simulink library "MS2G_Parts_Lib"  (R2016a)
settings: Solver=ode45  StartTime=0.0  StopTime=10.0  RelTol=1e-3
undefined symbols (not defined in the file or in its folder): Extr_Data_Link1Hole, Extr_Data_Link2Hole, Extr_Data_Ring, Local, X, Y, Z
libraries: sm_lib x58, MS2G_Parts_Lib x8
(part 1 of 2)
Description:
  | Copyright 2013-2016 The MathWorks, Inc.
settings Model: Creator=smiller  LastModifiedBy=smiller
settings DataIOCC: LimitDataPoints=on  SaveFormat=Array  SignalLoggingSaveFormat=ModelDataLogs
settings OptimizationCC: ExpressionDepthLimit=2147483647
settings DebuggingCC: UnderspecifiedInitializationDetection=Classic  MergeDetectMultiDrivingBlocksExec=none  SolverPrmCheckMsg=warning  FcnCallInpInsideContextMsg=EnableAllAsWarning  StateNameClashWarn=warning
settings HardwareCC: ProdBitPerPointer=32  ProdLargestAtomicFloat=None  ProdIntDivRoundTo=Undefined  ProdEndianess=Unspecified  ProdWordSize=32  ProdHWDeviceType=32-bit Generic
settings ModelReferenceCC: PropagateSignalLabelsOutOfModel=off
settings ConfigComp: CovModelRefEnable=Off

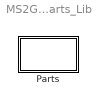
== system MS2G_Parts_Lib ==
  Parts : Subsystem

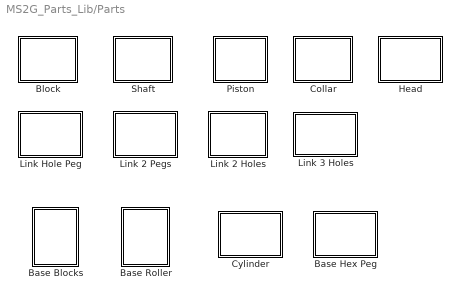
== system MS2G_Parts_Lib/Parts ==
  Base Blocks : Subsystem  mask(Base Blocks){block_length=6, block_width=16, block_height=16, shaft_radius=5, shaft_length=4.4, material_density=1000, material_color=[0 0.6 0.8], material_opacity=1}
      mask prompts: block_length "Length (cm)"; block_width "Width (cm)"; block_height "Height (cm)"; shaft_radius "Radius (cm)"; shaft_length "Length (cm)"; material_density "Density (kg/m^3)"; material_color "Color"; material_opacity "Opacity"
      mask help: Parameterized base with two blocks and a shaft.
      mask Display:
      | image(imread('Base_Blocks_IMAGE.jpg'));
      | port_label('RConn',1,'S');
      | port_label('LConn',1,'B');
  Base Hex Peg : Subsystem  mask(Four bar base body){R=3, T=0.5, rp=0.5, lp=1.5, clr=[0.4 0.4 0.4], img_file=sm_four_bar_base.png}
      mask prompts: R "Base radius (cm):"; T "Base thickeness (cm):"; rp "Peg radius (cm):"; lp "Peg length (cm):"; clr "Base color:"; img_file "Image file:"
      mask help: Base body on the crank side of the four bar mechanism
      mask Display:
      | image(imread('Base_Hex_Peg_IMAGE.jpg'));
      | port_label('LConn',1,'B');
      | port_label('RConn',1,'P');
  Base Roller : Subsystem  mask(Base Roller){roller_length=6, roller_radius=8, shaft_length=4.4, shaft_radius=5, material_density=1000, material_color=[0 0.6 0.8], material_opacity=1}
      mask prompts: roller_length "Length (cm)"; roller_radius "Radius (cm)"; shaft_length "Length (cm)"; shaft_radius "Radius (cm)"; material_density "Density (kg/m^3)"; material_color "Color"; material_opacity "Opacity"
      mask help: Parameterized roller with two wheels connected by a shaft.
      mask Display:
      | image(imread('Base_Roller_IMAGE.jpg'));
      | port_label('RConn',1,'S');
      | port_label('LConn',1,'B');
  Block : Subsystem  mask(Block){L=6, W=16, H=16, z_ori=Local +Z, rho=1000, clr=[0 0.6 0.8], opc=1}
      mask prompts: L "Length (cm):"; W "Width (cm):"; H "Height (cm):"; z_ori "Shaft orientation:"; rho "Shaft density (kg/m^3):"; clr "Link color:"; opc "Opacity:"
      mask help: Rectangular block. Ports are at the center of the faces normal to the local z-axis. Can be configured to have positive Z from B to F or from F to B.
      mask init:
      | if(z_ori == 2)
      |     z_ori = -1;
      | end
      mask TypeOptions z_ori: Local +Z | Local -Z
      mask Display:
      | image(imread('Block_IMAGE.jpg'));
      | port_label('LConn',1,'B');
      | port_label('RConn',1,'F');
  Collar : Subsystem  mask{collar_length=30, collar_radius=6.5, cylinder_length=20, cylinder_radius=6.5, cylinder_ori=Local +Z, material_density=1000, material_color=[0.5 0.5 0.5], material_opacity=1}
      mask prompts: collar_length "Length (cm):"; collar_radius "Radius (cm):"; cylinder_length "Length (cm):"; cylinder_radius "Radius (cm):"; cylinder_ori "Orientation (B to C):"; material_density "Density (kg/m^3):"; material_color "Color:"; material_opacity "Opacity:"
      mask init:
      | if(cylinder_ori == 2)
      |     cylinder_ori = -1;
      | end
      mask TypeOptions cylinder_ori: Local +Z | Local -Z
      mask Display:
      | image(imread('Actuator_Collar_IMAGE.jpg'));
      | port_label('LConn',1,'B');
      | port_label('RConn',1,'C');
  Cylinder : Subsystem  mask(Annular Cylinder){Ro=5, Ri=4, L=6, Ang_Sw=180, cyl_z=-4, cyl_theta=0, cyl_radius=18, rho=100, clr=[0.4 0.4 0.4], opc=0.5}
      mask prompts: Ro "Cylinder outer radius (cm)"; Ri "Cylinder inner radius (cm)"; L "Cylinder length (cm)"; Ang_Sw "Cylinder  sweep angle (deg)"; cyl_z "Z position (cm)"; cyl_theta "Theta (deg)"; cyl_radius "Radius (cm)"; rho "Density (kg/m^3)"; clr "Color"; opc "Opacity"
      mask Display:
      | image(imread('Cylinder_Half_IMAGE.jpg'));
      | port_label('LConn',1,'S')
      | port_label('RConn',1,'R')
  Head : Subsystem  mask(Piston Head){Ro=4, Ri=3, L=5, Rp=0.5, rho=100, clr=[0 1 0], opc=0.5}
      mask prompts: Ro "Cylinder outer radius (cm)"; Ri "Cylinder inner radius (cm)"; L "Cylinder length (cm)"; Rp "Pin radius (cm)"; rho "Density (kg/m^3)"; clr "Color"; opc "Opacity"
      mask help: Piston head with pin for rotating connection to rod. C port is aligned for translational motion in cylinder.
      mask Display:
      | image(imread('Piston_Peg_IMAGE.jpg'));
      | port_label('RConn',1,'C')
      | port_label('LConn',1,'P')
  Link 2 Holes : Subsystem  mask(Connector Link, 2 Holes){L=13, W=2, T=1, r=0.5, rho=10, clr=[0.6 0.6 0.0], opc=1}
      mask prompts: L "Link length (cm):"; W "Link width (cm):"; T "Link thickness (cm):"; r "Hole radius (cm):"; rho "Link density (kg/m^3):"; clr "Link color:"; opc "Opacity"
      mask help: Connector link with two holes. Ports are located at centers of holes, oriented such that Z is out of the hole, positive X is from L hole to R hole.
      mask Display:
      | image(imread('Link_Hole_Hole_IMAGE.jpg'));
      | port_label('LConn',1,'L');
      | port_label('RConn',1,'R');
  Link 2 Pegs : Subsystem  mask(Connector Link, 2 Pegs){L=4.5, W=2, T=0.5, r=0.5, z_ori_l=Local -Z, z_ori_r=Local -Z, Ro=1000, clr=[0.0 0.6 0.8], opc=1}
      mask prompts: L "Link length (cm):"; W "Link width (cm):"; T "Link thickness (cm):"; r "Peg radius (cm):"; z_ori_l "Peg Orientation, Left"; z_ori_r "Peg Orientation, Right"; Ro "Link density (kg/m^3):"; clr "Link color:"; opc "Opacity"
      mask help: Connector link with two pegs. The L and R ports are located at the outward face of each peg, and are oriented such that the Z-axis points along the axis of the peg, and positive X is from the left peg to the right peg. The pegs can be configured to be on the upper or lower side of the link.
      mask init:
      | if(z_ori_l == 2)
      |     z_ori_l = -1;
      | end
      | 
      | if(z_ori_r == 2)
      |     z_ori_r = -1;
      | end
      mask TypeOptions z_ori_l: Local +Z | Local -Z
      mask TypeOptions z_ori_r: Local +Z | Local -Z
      mask Display:
      | image(imread('Link_2Peg_IMAGE.jpg'));
      | port_label('LConn',1,'L');
      | port_label('RConn',1,'R');
  Link 3 Holes : Subsystem  mask(Connector Link, 2 Holes){L=240, W=15, T=4, r=5, rho=1000, clr_string=Yellow, opc=1}
      mask prompts: L "Link length (cm):"; W "Link width (cm):"; T "Link thickness (cm):"; r "Hole radius (cm):"; rho "Link density (kg/m^3):"; clr_string "Link color:"; opc "Opacity:"
      mask help: Connector link with two holes. Ports are located at centers of holes, oriented such that Z is out of the hole, positive X is from L hole to R hole.
      mask init:
      | imgfile='Link_3_Hole_Yellow_IMAGE.jpg';
      | if(strcmp(clr_string,'Yellow'))
      |     clr = [0.6 0.6 0.0];
      | else
      |     clr = [0.8 0.2 0.0];
      |     imgfile='Link_3_Hole_Red_IMAGE.jpg';
      | end
      mask TypeOptions clr_string: Yellow | Red
      mask Display:
      | image(imread(imgfile));
      | port_label('RConn',1,'F');
      | port_label('RConn',2,'C');
      | port_label('RConn',3,'R');
  Link Hole Peg : Subsystem  mask(Connector Link, Hole Peg){L=4.5, W=2, T=1.5, r=0.5, z_ori=Local +Z, Ro=1000, clr=[0.0 0.6 0.8], opc=1}
      mask prompts: L "Link length (cm):"; W "Link width (cm):"; T "Link thickness (cm):"; r "Peg/Hole radius (cm):"; z_ori "Peg Orientation:"; Ro "Link density (kg/m^3):"; clr "Link color:"; opc "Opacity"
      mask help: Connector Link with one hole and one peg. The H port is at the center of the hole. The P port is at the outward face of the peg. Frames are oriented such that Z points out of the hole, positive X is from the hole to the peg. The peg can be placed on the upper or lower side of the link.
      mask init:
      | if(z_ori == 2)
      |     z_ori = -1;
      | end
      mask TypeOptions z_ori: Local +Z | Local -Z
      mask Display:
      | image(imread('Link_Hole_Peg_IMAGE.jpg'));
      | port_label('LConn',1,'H');
      | port_label('RConn',1,'P');
  Piston : Subsystem
      mask Display:
      | image(imread('Piston_Shaft_IMAGE.jpg'));
      | port_label('RConn',1,'P');
      | port_label('LConn',1,'R');
  Shaft : Subsystem  mask(Cylindrical Shaft){L=10, r=5, theta=0, z_ori=Local -Z, Ro=1000, clr=[0.0 0.6 0.8], opc=1}
      mask prompts: L "Length (cm):"; r "Radius (cm):"; theta "Twist (deg)"; z_ori "Orientation (B to F)"; Ro "Density (kg/m^3):"; clr "Color:"; opc "Opacity"
      mask help: Cylindrical shaft. Ports are at shaft ends, and oriented such that the Z-axis is between the ports. Can be configured to have positive Z from B to F or from F to B.
      mask init:
      | if(z_ori == 2)
      |     z_ori = -1;
      | end
      mask TypeOptions z_ori: Local +Z | Local -Z
      mask Display:
      | image(imread('Shaft_IMAGE.jpg'));
      | port_label('LConn',1,'B');
      | port_label('RConn',1,'F');

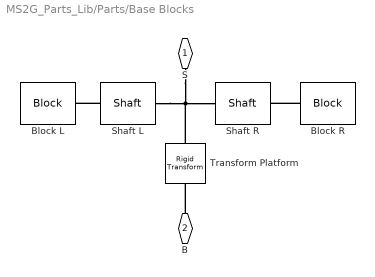
== system MS2G_Parts_Lib/Parts/Base Blocks ==
  Block L : MS2G_Parts_Lib/Parts/Block  L=block_length  W=block_width  H=block_height  z_ori=Local -Z  rho=material_density  clr=material_color  opc=material_opacity
  Block R : MS2G_Parts_Lib/Parts/Block  L=block_length  W=block_width  H=block_height  z_ori=Local +Z  rho=material_density  clr=material_color  opc=material_opacity
  Shaft L : MS2G_Parts_Lib/Parts/Shaft  L=shaft_length/2  r=shaft_radius  theta=0  z_ori=Local -Z  Ro=material_density  clr=material_color  opc=material_opacity
  Shaft R : MS2G_Parts_Lib/Parts/Shaft  L=shaft_length/2  r=shaft_radius  theta=0  z_ori=Local +Z  Ro=material_density  clr=material_color  opc=material_opacity
  Transform Platform : sm_lib/Frames and Transforms/Rigid Transform  TranslationMethod=Cartesian  TranslationLengthUnit=cm  TranslationStandardAxis=-Y  TranslationStandardOffset=1  TranslationCartesianOffset=[0 -block_height/2 0]  TranslationROffset=0  TranslationROffsetUnits=m  TranslationZOffset=0  TranslationZOffsetUnits=m  TranslationThetaOffset=0  TranslationThetaOffsetUnits=deg  RotationMethod=None  RotationAngleUnits=deg  RotationStandardAxis=+Y  RotationAngle=0  RotationArbitraryAxis=[0 0 1]  FollAlignAxisA=+X  BaseAlignAxisA=+Y  FollAlignAxisB=+Y  BaseAlignAxisB=+Z  RotationSequenceAxes=FollowerAxes  RotationSequence=XYX  RotationSequenceAngles=[0 0 0]  RotationSequenceAnglesUnits=deg  RotationMatrix=[1 0 0; 0 1 0; 0 0 1]
  S : PMIOPort  Port=1  Side=Right
  B : PMIOPort  Port=2  Side=Left
  connections:
  S/RConn1 -- Transform Platform/LConn1 -- Shaft R/LConn1 -- Shaft L/LConn1
  B/RConn1 -- Transform Platform/RConn1
  Block R/LConn1 -- Shaft R/RConn1
  Shaft L/RConn1 -- Block L/LConn1

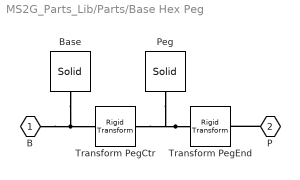
== system MS2G_Parts_Lib/Parts/Base Hex Peg ==
  Base : sm_lib/Body Elements/Solid  InertiaType=CalculateFromGeometry  Mass=1  MassUnits=kg  CenterOfMass=[0 0 0]  CenterOfMassUnits=m  MomentsOfInertia=[1 1 1]  MomentsOfInertiaUnits=kg*m^2  ProductsOfInertia=[0 0 0]  ProductsOfInertiaUnits=kg*m^2  DensityBased=on  Density=1  DensityUnits=kg/(m^3)  DoExposeReferenceFrame=on  SerializedFrames=<Frames/>  GraphicType=FromGeometry  MarkerShape=Sphere  MarkerSize=1  MarkerSizeUnits=m  GraphicVisPropType=SimpleVisualProperties  GraphicDiffuseColor=clr  GraphicSpecularColor=[0.2 0.2 0.2]  GraphicAmbientColor=[0.5 0.5 0.5]  GraphicEmissiveColor=[0.1 0.1 0.1]  GraphicShininess=24.0  GraphicOpacity=1  GeometryShape=RegularExtrusion  RectangleSize=[1 1]  RectangleSizeUnits=m  BrickDimensions=[10 5 T]  BrickDimensionUnits=cm  CylinderRadius=R  CylinderRadiusUnits=cm  CylinderLength=T  CylinderLengthUnits=cm  SphereRadius=1  SphereRadiusUnits=m  EllipsoidRadii=[1 1 1]  EllipsoidRadiiUnits=m  ExtrusionCrossSection=[1 1; -1 1; -1 -1; 1 -1]  ExtrusionCrossSectionUnits=m  ExtrusionLength=T  ExtrusionLengthUnits=cm  PolygonNumSides=6  PolygonOuterRadius=R  PolygonOuterRadiusUnits=cm  ExtGeomFileType=STEP  ExtGeomFileUnits=m  RevolutionCrossSection=[1 1; 1 -1; 2 -1; 2 1]  RevolutionCrossSectionUnits=m  RevolutionExtent=Full  RevolutionAngle=180  RevolutionAngleUnits=deg
  Peg : sm_lib/Body Elements/Solid  InertiaType=CalculateFromGeometry  Mass=1  MassUnits=kg  CenterOfMass=[0 0 0]  CenterOfMassUnits=m  MomentsOfInertia=[1 1 1]  MomentsOfInertiaUnits=kg*m^2  ProductsOfInertia=[0 0 0]  ProductsOfInertiaUnits=kg*m^2  DensityBased=on  Density=1  DensityUnits=kg/m^3  DoExposeReferenceFrame=on  SerializedFrames=<Frames/>  GraphicType=FromGeometry  MarkerShape=Sphere  MarkerSize=1  MarkerSizeUnits=m  GraphicVisPropType=SimpleVisualProperties  GraphicDiffuseColor=clr  GraphicSpecularColor=[0.2 0.2 0.2]  GraphicAmbientColor=[0.5 0.5 0.5]  GraphicEmissiveColor=[0.1 0.1 0.1]  GraphicShininess=24.0  GraphicOpacity=1  GeometryShape=Cylinder  RectangleSize=[1 1]  RectangleSizeUnits=m  BrickDimensions=[1 1 1]  BrickDimensionUnits=m  CylinderRadius=rp  CylinderRadiusUnits=cm  CylinderLength=lp  CylinderLengthUnits=cm  SphereRadius=1  SphereRadiusUnits=m  EllipsoidRadii=[1 1 1]  EllipsoidRadiiUnits=m  ExtrusionCrossSection=[1 1; -1 1; -1 -1; 1 -1]  ExtrusionCrossSectionUnits=m  ExtrusionLength=1  ExtrusionLengthUnits=m  PolygonNumSides=1  PolygonOuterRadius=1  PolygonOuterRadiusUnits=m  ExtGeomFileType=STEP  ExtGeomFileUnits=m  RevolutionCrossSection=[1 1; 1 -1; 2 -1; 2 1]  RevolutionCrossSectionUnits=m  RevolutionExtent=Full  RevolutionAngle=180  RevolutionAngleUnits=deg
  Transform PegCtr : sm_lib/Frames and Transforms/Rigid Transform  TranslationMethod=StandardAxis  TranslationLengthUnit=cm  TranslationStandardAxis=-Z  TranslationStandardOffset=(T+lp)/2  TranslationCartesianOffset=[0 0 0]  TranslationROffset=0  TranslationROffsetUnits=m  TranslationZOffset=0  TranslationZOffsetUnits=m  TranslationThetaOffset=0  TranslationThetaOffsetUnits=deg  RotationMethod=None  RotationAngleUnits=deg  RotationStandardAxis=+Z  RotationAngle=0  RotationArbitraryAxis=[0 0 1]  FollAlignAxisA=+X  BaseAlignAxisA=+Y  FollAlignAxisB=+Y  BaseAlignAxisB=+Z  RotationSequenceAxes=FollowerAxes  RotationSequence=XYX  RotationSequenceAngles=[0 0 0]  RotationSequenceAnglesUnits=deg  RotationMatrix=[1 0 0; 0 1 0; 0 0 1]
  Transform PegEnd : sm_lib/Frames and Transforms/Rigid Transform  TranslationMethod=StandardAxis  TranslationLengthUnit=cm  TranslationStandardAxis=-Z  TranslationStandardOffset=lp/2  TranslationCartesianOffset=[0 0 0]  TranslationROffset=0  TranslationROffsetUnits=m  TranslationZOffset=0  TranslationZOffsetUnits=m  TranslationThetaOffset=0  TranslationThetaOffsetUnits=deg  RotationMethod=None  RotationAngleUnits=deg  RotationStandardAxis=+Z  RotationAngle=0  RotationArbitraryAxis=[0 0 1]  FollAlignAxisA=+X  BaseAlignAxisA=+Y  FollAlignAxisB=+Y  BaseAlignAxisB=+Z  RotationSequenceAxes=FollowerAxes  RotationSequence=XYX  RotationSequenceAngles=[0 0 0]  RotationSequenceAnglesUnits=deg  RotationMatrix=[1 0 0; 0 1 0; 0 0 1]
  B : PMIOPort  Port=1  Side=Left
  P : PMIOPort  Port=2  Side=Right
  connections:
  P/RConn1 -- Transform PegEnd/RConn1
  Transform PegEnd/LConn1 -- Peg/RConn1 -- Transform PegCtr/RConn1
  Base/RConn1 -- B/RConn1 -- Transform PegCtr/LConn1

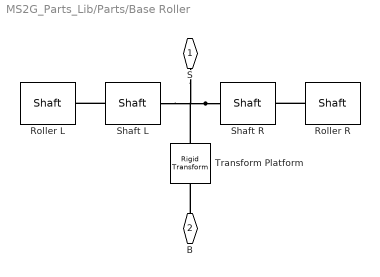
== system MS2G_Parts_Lib/Parts/Base Roller ==
  Roller L : MS2G_Parts_Lib/Parts/Shaft  L=roller_length  r=roller_radius  theta=0  z_ori=Local -Z  Ro=material_density  clr=material_color  opc=material_opacity
  Roller R : MS2G_Parts_Lib/Parts/Shaft  L=roller_length  r=roller_radius  theta=0  z_ori=Local +Z  Ro=material_density  clr=material_color  opc=material_opacity
  Shaft L : MS2G_Parts_Lib/Parts/Shaft  L=shaft_length/2  r=shaft_radius  theta=0  z_ori=Local -Z  Ro=material_density  clr=material_color  opc=material_opacity
  Shaft R : MS2G_Parts_Lib/Parts/Shaft  L=shaft_length/2  r=shaft_radius  theta=0  z_ori=Local +Z  Ro=material_density  clr=material_color  opc=material_opacity
  Transform Platform : sm_lib/Frames and Transforms/Rigid Transform  TranslationMethod=StandardAxis  TranslationLengthUnit=cm  TranslationStandardAxis=-Y  TranslationStandardOffset=roller_radius  TranslationCartesianOffset=[0 0 0]  TranslationROffset=0  TranslationROffsetUnits=m  TranslationZOffset=0  TranslationZOffsetUnits=m  TranslationThetaOffset=0  TranslationThetaOffsetUnits=deg  RotationMethod=StandardAxis  RotationAngleUnits=deg  RotationStandardAxis=+Y  RotationAngle=90  RotationArbitraryAxis=[0 0 1]  FollAlignAxisA=+X  BaseAlignAxisA=+Y  FollAlignAxisB=+Y  BaseAlignAxisB=+Z  RotationSequenceAxes=FollowerAxes  RotationSequence=XYX  RotationSequenceAngles=[0 0 0]  RotationSequenceAnglesUnits=deg  RotationMatrix=[1 0 0; 0 1 0; 0 0 1]
  S : PMIOPort  Port=1  Side=Right
  B : PMIOPort  Port=2  Side=Left
  connections:
  B/RConn1 -- Transform Platform/RConn1
  Shaft R/LConn1 -- Transform Platform/LConn1 -- Shaft L/LConn1 -- S/RConn1
  Roller R/LConn1 -- Shaft R/RConn1
  Shaft L/RConn1 -- Roller L/LConn1

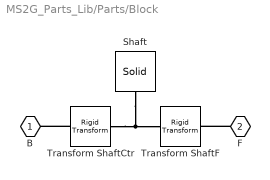
== system MS2G_Parts_Lib/Parts/Block ==
  Shaft : sm_lib/Body Elements/Solid  InertiaType=CalculateFromGeometry  Mass=1  MassUnits=kg  CenterOfMass=[0 0 0]  CenterOfMassUnits=m  MomentsOfInertia=[1 1 1]  MomentsOfInertiaUnits=kg*m^2  ProductsOfInertia=[0 0 0]  ProductsOfInertiaUnits=kg*m^2  DensityBased=on  Density=rho  DensityUnits=kg/m^3  DoExposeReferenceFrame=on  SerializedFrames=<Frames/>  GraphicType=FromGeometry  MarkerShape=Sphere  MarkerSize=1  MarkerSizeUnits=m  GraphicVisPropType=SimpleVisualProperties  GraphicDiffuseColor=clr  GraphicSpecularColor=[0.2 0.2 0.2]  GraphicAmbientColor=[0.5 0.5 0.5]  GraphicEmissiveColor=[0.1 0.1 0.1]  GraphicShininess=24.0  GraphicOpacity=opc  GeometryShape=Brick  RectangleSize=[1 1]  RectangleSizeUnits=m  BrickDimensions=[W H L]  BrickDimensionUnits=cm  CylinderRadius=1  CylinderRadiusUnits=cm  CylinderLength=1  CylinderLengthUnits=cm  SphereRadius=1  SphereRadiusUnits=m  EllipsoidRadii=[1 1 1]  EllipsoidRadiiUnits=m  ExtrusionCrossSection=[1 1; -1 1; -1 -1; 1 -1]  ExtrusionCrossSectionUnits=m  ExtrusionLength=1  ExtrusionLengthUnits=m  PolygonNumSides=1  PolygonOuterRadius=1  PolygonOuterRadiusUnits=m  ExtGeomFileType=STEP  ExtGeomFileUnits=m  RevolutionCrossSection=[1 1; 1 -1; 2 -1; 2 1]  RevolutionCrossSectionUnits=m  RevolutionExtent=Full  RevolutionAngle=180  RevolutionAngleUnits=deg
  Transform ShaftCtr : sm_lib/Frames and Transforms/Rigid Transform  TranslationMethod=Cartesian  TranslationLengthUnit=cm  TranslationStandardAxis=+Z  TranslationStandardOffset=0  TranslationCartesianOffset=[0 0 L/2]*z_ori  TranslationROffset=0  TranslationROffsetUnits=m  TranslationZOffset=0  TranslationZOffsetUnits=m  TranslationThetaOffset=0  TranslationThetaOffsetUnits=deg  RotationMethod=None  RotationAngleUnits=deg  RotationStandardAxis=+Z  RotationAngle=0  RotationArbitraryAxis=[0 0 1]  FollAlignAxisA=+X  BaseAlignAxisA=+Y  FollAlignAxisB=+Y  BaseAlignAxisB=+Z  RotationSequenceAxes=FollowerAxes  RotationSequence=XYX  RotationSequenceAngles=[0 0 0]  RotationSequenceAnglesUnits=deg  RotationMatrix=[1 0 0; 0 1 0; 0 0 1]
  Transform ShaftF : sm_lib/Frames and Transforms/Rigid Transform  TranslationMethod=Cartesian  TranslationLengthUnit=cm  TranslationStandardAxis=+Z  TranslationStandardOffset=0  TranslationCartesianOffset=[0 0 L/2]*z_ori  TranslationROffset=0  TranslationROffsetUnits=m  TranslationZOffset=0  TranslationZOffsetUnits=m  TranslationThetaOffset=0  TranslationThetaOffsetUnits=deg  RotationMethod=None  RotationAngleUnits=deg  RotationStandardAxis=+Z  RotationAngle=0  RotationArbitraryAxis=[0 0 1]  FollAlignAxisA=+X  BaseAlignAxisA=+Y  FollAlignAxisB=+Y  BaseAlignAxisB=+Z  RotationSequenceAxes=FollowerAxes  RotationSequence=XYX  RotationSequenceAngles=[0 0 0]  RotationSequenceAnglesUnits=deg  RotationMatrix=[1 0 0; 0 1 0; 0 0 1]
  B : PMIOPort  Port=1  Side=Left
  F : PMIOPort  Port=2  Side=Right
  connections:
  Transform ShaftCtr/RConn1 -- Transform ShaftF/LConn1 -- Shaft/RConn1
  F/RConn1 -- Transform ShaftF/RConn1
  Transform ShaftCtr/LConn1 -- B/RConn1

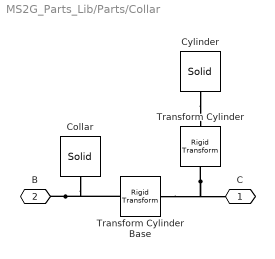
== system MS2G_Parts_Lib/Parts/Collar ==
  Collar : sm_lib/Body Elements/Solid  InertiaType=CalculateFromGeometry  Mass=1  MassUnits=kg  CenterOfMass=[0 0 0]  CenterOfMassUnits=m  MomentsOfInertia=[1 1 1]  MomentsOfInertiaUnits=kg*m^2  ProductsOfInertia=[0 0 0]  ProductsOfInertiaUnits=kg*m^2  DensityBased=on  Density=material_density  DensityUnits=kg/(m^3)  DoExposeReferenceFrame=on  SerializedFrames=<Frames/>  GraphicType=FromGeometry  MarkerShape=Sphere  MarkerSize=10  MarkerSizeUnits=m  GraphicVisPropType=SimpleVisualProperties  GraphicDiffuseColor=material_color  GraphicSpecularColor=[0.5 0.5 0.5 1.0]  GraphicAmbientColor=[0.15 0.15 0.15 1.0]  GraphicEmissiveColor=[0.0 0.0 0.0 1.0]  GraphicShininess=75  GraphicOpacity=material_opacity  GeometryShape=GeneralExtrusion  RectangleSize=[1 1]  RectangleSizeUnits=m  BrickDimensions=[10 10 100]  BrickDimensionUnits=cm  CylinderRadius=1  CylinderRadiusUnits=cm  CylinderLength=1  CylinderLengthUnits=cm  SphereRadius=1  SphereRadiusUnits=m  EllipsoidRadii=[1 1 1]  EllipsoidRadiiUnits=m  ExtrusionCrossSection=Extr_Data_Ring(collar_radius,collar_radius*0.9,0,360)  ExtrusionCrossSectionUnits=cm  ExtrusionLength=collar_length  ExtrusionLengthUnits=cm  PolygonNumSides=3  PolygonOuterRadius=1  PolygonOuterRadiusUnits=m  ExtGeomFileType=STEP  ExtGeomFileUnits=m  RevolutionCrossSection=[1 1; 1 -1; 2 -1; 2 1]  RevolutionCrossSectionUnits=m  RevolutionExtent=Full  RevolutionAngle=180  RevolutionAngleUnits=deg
  Cylinder : sm_lib/Body Elements/Solid  InertiaType=CalculateFromGeometry  Mass=1  MassUnits=kg  CenterOfMass=[0 0 0]  CenterOfMassUnits=m  MomentsOfInertia=[1 1 1]  MomentsOfInertiaUnits=kg*m^2  ProductsOfInertia=[0 0 0]  ProductsOfInertiaUnits=kg*m^2  DensityBased=on  Density=material_density  DensityUnits=kg/(m^3)  DoExposeReferenceFrame=on  SerializedFrames=<Frames/>  GraphicType=FromGeometry  MarkerShape=Sphere  MarkerSize=10  MarkerSizeUnits=m  GraphicVisPropType=SimpleVisualProperties  GraphicDiffuseColor=material_color  GraphicSpecularColor=[0.5 0.5 0.5 1.0]  GraphicAmbientColor=[0.15 0.15 0.15 1.0]  GraphicEmissiveColor=[0.0 0.0 0.0 1.0]  GraphicShininess=75  GraphicOpacity=material_opacity  GeometryShape=GeneralExtrusion  RectangleSize=[1 1]  RectangleSizeUnits=m  BrickDimensions=[10 10 100]  BrickDimensionUnits=cm  CylinderRadius=1  CylinderRadiusUnits=cm  CylinderLength=1  CylinderLengthUnits=cm  SphereRadius=1  SphereRadiusUnits=m  EllipsoidRadii=[1 1 1]  EllipsoidRadiiUnits=m  ExtrusionCrossSection=Extr_Data_Ring(cylinder_radius,cylinder_radius*0.9,0,360)  ExtrusionCrossSectionUnits=cm  ExtrusionLength=cylinder_length  ExtrusionLengthUnits=cm  PolygonNumSides=3  PolygonOuterRadius=1  PolygonOuterRadiusUnits=m  ExtGeomFileType=STEP  ExtGeomFileUnits=m  RevolutionCrossSection=[1 1; 1 -1; 2 -1; 2 1]  RevolutionCrossSectionUnits=m  RevolutionExtent=Full  RevolutionAngle=180  RevolutionAngleUnits=deg
  Transform Cylinder : sm_lib/Frames and Transforms/Rigid Transform  TranslationMethod=StandardAxis  TranslationLengthUnit=cm  TranslationStandardAxis=+Z  TranslationStandardOffset=cylinder_length/2*cylinder_ori  TranslationCartesianOffset=[0 0 0]  TranslationROffset=0  TranslationROffsetUnits=m  TranslationZOffset=0  TranslationZOffsetUnits=m  TranslationThetaOffset=0  TranslationThetaOffsetUnits=deg  RotationMethod=None  RotationAngleUnits=deg  RotationStandardAxis=+Y  RotationAngle=0  RotationArbitraryAxis=[0 0 1]  FollAlignAxisA=+X  BaseAlignAxisA=+Y  FollAlignAxisB=+Y  BaseAlignAxisB=+Z  RotationSequenceAxes=FollowerAxes  RotationSequence=XYX  RotationSequenceAngles=[0 0 0]  RotationSequenceAnglesUnits=deg  RotationMatrix=[1 0 0; 0 1 0; 0 0 1]
  Transform Cylinder Base : sm_lib/Frames and Transforms/Rigid Transform  TranslationMethod=None  TranslationLengthUnit=m  TranslationStandardAxis=+Z  TranslationStandardOffset=0  TranslationCartesianOffset=[0 0 0]  TranslationROffset=0  TranslationROffsetUnits=m  TranslationZOffset=0  TranslationZOffsetUnits=m  TranslationThetaOffset=0  TranslationThetaOffsetUnits=deg  RotationMethod=StandardAxis  RotationAngleUnits=deg  RotationStandardAxis=-Y  RotationAngle=90  RotationArbitraryAxis=[0 0 1]  FollAlignAxisA=+X  BaseAlignAxisA=+Y  FollAlignAxisB=+Y  BaseAlignAxisB=+Z  RotationSequenceAxes=FollowerAxes  RotationSequence=XYX  RotationSequenceAngles=[0 0 0]  RotationSequenceAnglesUnits=deg  RotationMatrix=[1 0 0; 0 1 0; 0 0 1]
  C : PMIOPort  Port=1  Side=Right
  B : PMIOPort  Port=2  Side=Left
  connections:
  Transform Cylinder/LConn1 -- Transform Cylinder Base/RConn1 -- C/RConn1
  Cylinder/RConn1 -- Transform Cylinder/RConn1
  B/RConn1 -- Collar/RConn1 -- Transform Cylinder Base/LConn1

== system MS2G_Parts_Lib/Parts/Cylinder ==
  Ring : sm_lib/Body Elements/Solid  InertiaType=CalculateFromGeometry  Mass=1  MassUnits=kg  CenterOfMass=[0 0 0]  CenterOfMassUnits=m  MomentsOfInertia=[1 1 1]  MomentsOfInertiaUnits=kg*m^2  ProductsOfInertia=[0 0 0]  ProductsOfInertiaUnits=kg*m^2  DensityBased=on  Density=rho  DensityUnits=kg/(m^3)  DoExposeReferenceFrame=on  SerializedFrames=<Frames/>  GraphicType=FromGeometry  MarkerShape=Sphere  MarkerSize=10  MarkerSizeUnits=m  GraphicVisPropType=SimpleVisualProperties  GraphicDiffuseColor=clr  GraphicSpecularColor=[0.5 0.5 0.5 1.0]  GraphicAmbientColor=[0.5 0.0 0.0 1.0]  GraphicEmissiveColor=[0.0 0.0 0.0 1.0]  GraphicShininess=75  GraphicOpacity=opc  GeometryShape=GeneralExtrusion  RectangleSize=[1 1]  RectangleSizeUnits=m  BrickDimensions=[1 1 1]  BrickDimensionUnits=m  CylinderRadius=1  CylinderRadiusUnits=m  CylinderLength=1  CylinderLengthUnits=m  SphereRadius=1  SphereRadiusUnits=m  EllipsoidRadii=[1 1 1]  EllipsoidRadiiUnits=m  ExtrusionCrossSection=Extr_Data_Ring(Ro,Ri,0,Ang_Sw)  ExtrusionCrossSectionUnits=cm  ExtrusionLength=L  ExtrusionLengthUnits=cm  PolygonNumSides=3  PolygonOuterRadius=1  PolygonOuterRadiusUnits=m  ExtGeomFileType=STEP  ExtGeomFileUnits=m  RevolutionCrossSection=[1 1; 1 -1; 2 -1; 2 1]  RevolutionCrossSectionUnits=m  RevolutionExtent=Full  RevolutionAngle=180  RevolutionAngleUnits=deg
  Transform Centerline : sm_lib/Frames and Transforms/Rigid Transform  TranslationMethod=None  TranslationLengthUnit=cm  TranslationStandardAxis=+X  TranslationStandardOffset=0  TranslationCartesianOffset=[0 0 0]  TranslationROffset=0  TranslationROffsetUnits=cm  TranslationZOffset=0  TranslationZOffsetUnits=cm  TranslationThetaOffset=0  TranslationThetaOffsetUnits=deg  RotationMethod=StandardAxis  RotationAngleUnits=deg  RotationStandardAxis=+Z  RotationAngle=cyl_theta  RotationArbitraryAxis=[0 0 1]  FollAlignAxisA=+X  BaseAlignAxisA=+Y  FollAlignAxisB=+Y  BaseAlignAxisB=+Z  RotationSequenceAxes=FollowerAxes  RotationSequence=XYX  RotationSequenceAngles=[0 0 0]  RotationSequenceAnglesUnits=deg  RotationMatrix=[1 0 0; 0 1 0; 0 0 1]
  Transform Ring : sm_lib/Frames and Transforms/Rigid Transform  TranslationMethod=Cylindrical  TranslationLengthUnit=cm  TranslationStandardAxis=+X  TranslationStandardOffset=0  TranslationCartesianOffset=[0 0 0]  TranslationROffset=cyl_radius  TranslationROffsetUnits=cm  TranslationZOffset=cyl_z  TranslationZOffsetUnits=cm  TranslationThetaOffset=0  TranslationThetaOffsetUnits=deg  RotationMethod=StandardAxis  RotationAngleUnits=deg  RotationStandardAxis=+Y  RotationAngle=90  RotationArbitraryAxis=[0 0 1]  FollAlignAxisA=+X  BaseAlignAxisA=+Y  FollAlignAxisB=+Y  BaseAlignAxisB=+Z  RotationSequenceAxes=FollowerAxes  RotationSequence=XYX  RotationSequenceAngles=[0 0 0]  RotationSequenceAnglesUnits=deg  RotationMatrix=[1 0 0; 0 1 0; 0 0 1]
  S : PMIOPort  Port=1  Side=Left
  R : PMIOPort  Port=2  Side=Right
  connections:
  Transform Centerline/RConn1 -- Transform Ring/LConn1
  Transform Centerline/LConn1 -- S/RConn1
  Transform Ring/RConn1 -- R/RConn1 -- Ring/RConn1

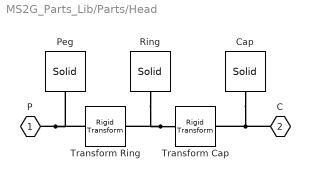
== system MS2G_Parts_Lib/Parts/Head ==
  Cap : sm_lib/Body Elements/Solid  InertiaType=CalculateFromGeometry  Mass=1  MassUnits=kg  CenterOfMass=[0 0 0]  CenterOfMassUnits=m  MomentsOfInertia=[1 1 1]  MomentsOfInertiaUnits=kg*m^2  ProductsOfInertia=[0 0 0]  ProductsOfInertiaUnits=kg*m^2  DensityBased=on  Density=1  DensityUnits=kg/(m^3)  DoExposeReferenceFrame=on  SerializedFrames=<Frames/>  GraphicType=FromGeometry  MarkerShape=Sphere  MarkerSize=1  MarkerSizeUnits=m  GraphicVisPropType=SimpleVisualProperties  GraphicDiffuseColor=clr  GraphicSpecularColor=[0.2 0.2 0.2]  GraphicAmbientColor=[0.5 0.5 0.5]  GraphicEmissiveColor=[0.1 0.1 0.1]  GraphicShininess=24.0  GraphicOpacity=opc  GeometryShape=Cylinder  RectangleSize=[1 1]  RectangleSizeUnits=m  BrickDimensions=[1 1 1]  BrickDimensionUnits=m  CylinderRadius=Ro  CylinderRadiusUnits=cm  CylinderLength=(Ro-Ri)  CylinderLengthUnits=cm  SphereRadius=1  SphereRadiusUnits=m  EllipsoidRadii=[1 1 1]  EllipsoidRadiiUnits=m  ExtrusionCrossSection=[1 1; -1 1; -1 -1; 1 -1]  ExtrusionCrossSectionUnits=m  ExtrusionLength=1  ExtrusionLengthUnits=m  PolygonNumSides=1  PolygonOuterRadius=1  PolygonOuterRadiusUnits=m  ExtGeomFileType=STEP  ExtGeomFileUnits=m  RevolutionCrossSection=[1 1; 1 -1; 2 -1; 2 1]  RevolutionCrossSectionUnits=m  RevolutionExtent=Full  RevolutionAngle=180  RevolutionAngleUnits=deg
  Peg : sm_lib/Body Elements/Solid  InertiaType=CalculateFromGeometry  Mass=1  MassUnits=kg  CenterOfMass=[0 0 0]  CenterOfMassUnits=m  MomentsOfInertia=[1 1 1]  MomentsOfInertiaUnits=kg*m^2  ProductsOfInertia=[0 0 0]  ProductsOfInertiaUnits=kg*m^2  DensityBased=on  Density=1  DensityUnits=kg/(m^3)  DoExposeReferenceFrame=on  SerializedFrames=<Frames/>  GraphicType=FromGeometry  MarkerShape=Sphere  MarkerSize=1  MarkerSizeUnits=m  GraphicVisPropType=SimpleVisualProperties  GraphicDiffuseColor=clr  GraphicSpecularColor=[0.2 0.2 0.2]  GraphicAmbientColor=[0.5 0.5 0.5]  GraphicEmissiveColor=[0.1 0.1 0.1]  GraphicShininess=24.0  GraphicOpacity=1  GeometryShape=Cylinder  RectangleSize=[1 1]  RectangleSizeUnits=m  BrickDimensions=[1 1 1]  BrickDimensionUnits=m  CylinderRadius=Rp  CylinderRadiusUnits=cm  CylinderLength=(Ro+Ri)  CylinderLengthUnits=cm  SphereRadius=1  SphereRadiusUnits=m  EllipsoidRadii=[1 1 1]  EllipsoidRadiiUnits=m  ExtrusionCrossSection=[1 1; -1 1; -1 -1; 1 -1]  ExtrusionCrossSectionUnits=m  ExtrusionLength=1  ExtrusionLengthUnits=m  PolygonNumSides=1  PolygonOuterRadius=1  PolygonOuterRadiusUnits=m  ExtGeomFileType=STEP  ExtGeomFileUnits=m  RevolutionCrossSection=[1 1; 1 -1; 2 -1; 2 1]  RevolutionCrossSectionUnits=m  RevolutionExtent=Full  RevolutionAngle=180  RevolutionAngleUnits=deg
  Ring : sm_lib/Body Elements/Solid  InertiaType=CalculateFromGeometry  Mass=1  MassUnits=kg  CenterOfMass=[0 0 0]  CenterOfMassUnits=m  MomentsOfInertia=[1 1 1]  MomentsOfInertiaUnits=kg*m^2  ProductsOfInertia=[0 0 0]  ProductsOfInertiaUnits=kg*m^2  DensityBased=on  Density=rho  DensityUnits=kg/(m^3)  DoExposeReferenceFrame=on  SerializedFrames=<Frames/>  GraphicType=FromGeometry  MarkerShape=Sphere  MarkerSize=10  MarkerSizeUnits=m  GraphicVisPropType=SimpleVisualProperties  GraphicDiffuseColor=clr  GraphicSpecularColor=[0.5 0.5 0.5 1.0]  GraphicAmbientColor=[0.5 0.0 0.0 1.0]  GraphicEmissiveColor=[0.0 0.0 0.0 1.0]  GraphicShininess=75  GraphicOpacity=opc  GeometryShape=GeneralExtrusion  RectangleSize=[1 1]  RectangleSizeUnits=m  BrickDimensions=[1 1 1]  BrickDimensionUnits=m  CylinderRadius=1  CylinderRadiusUnits=m  CylinderLength=1  CylinderLengthUnits=m  SphereRadius=1  SphereRadiusUnits=m  EllipsoidRadii=[1 1 1]  EllipsoidRadiiUnits=m  ExtrusionCrossSection=Extr_Data_Ring(Ro,Ri,0,360)  ExtrusionCrossSectionUnits=cm  ExtrusionLength=L  ExtrusionLengthUnits=cm  PolygonNumSides=3  PolygonOuterRadius=1  PolygonOuterRadiusUnits=m  ExtGeomFileType=STEP  ExtGeomFileUnits=m  RevolutionCrossSection=[1 1; 1 -1; 2 -1; 2 1]  RevolutionCrossSectionUnits=m  RevolutionExtent=Full  RevolutionAngle=180  RevolutionAngleUnits=deg
  Transform Cap : sm_lib/Frames and Transforms/Rigid Transform  TranslationMethod=StandardAxis  TranslationLengthUnit=cm  TranslationStandardAxis=+Z  TranslationStandardOffset=L/2+(Ro-Ri)/2  TranslationCartesianOffset=[0 0 0]  TranslationROffset=0  TranslationROffsetUnits=m  TranslationZOffset=0  TranslationZOffsetUnits=m  TranslationThetaOffset=0  TranslationThetaOffsetUnits=deg  RotationMethod=None  RotationAngleUnits=deg  RotationStandardAxis=+Z  RotationAngle=0  RotationArbitraryAxis=[0 0 1]  FollAlignAxisA=+X  BaseAlignAxisA=+Y  FollAlignAxisB=+Y  BaseAlignAxisB=+Z  RotationSequenceAxes=FollowerAxes  RotationSequence=XYX  RotationSequenceAngles=[0 0 0]  RotationSequenceAnglesUnits=deg  RotationMatrix=[1 0 0; 0 1 0; 0 0 1]
  Transform Ring : sm_lib/Frames and Transforms/Rigid Transform  TranslationMethod=None  TranslationLengthUnit=cm  TranslationStandardAxis=+X  TranslationStandardOffset=0  TranslationCartesianOffset=[0 0 0]  TranslationROffset=0  TranslationROffsetUnits=m  TranslationZOffset=0  TranslationZOffsetUnits=m  TranslationThetaOffset=0  TranslationThetaOffsetUnits=deg  RotationMethod=StandardAxis  RotationAngleUnits=deg  RotationStandardAxis=+Y  RotationAngle=90  RotationArbitraryAxis=[0 0 1]  FollAlignAxisA=+X  BaseAlignAxisA=+Y  FollAlignAxisB=+Y  BaseAlignAxisB=+Z  RotationSequenceAxes=FollowerAxes  RotationSequence=XYX  RotationSequenceAngles=[0 0 0]  RotationSequenceAnglesUnits=deg  RotationMatrix=[1 0 0; 0 1 0; 0 0 1]
  P : PMIOPort  Port=1  Side=Left
  C : PMIOPort  Port=2  Side=Right
  connections:
  C/RConn1 -- Transform Cap/RConn1 -- Cap/RConn1
  Transform Cap/LConn1 -- Transform Ring/RConn1 -- Ring/RConn1
  P/RConn1 -- Transform Ring/LConn1 -- Peg/RConn1

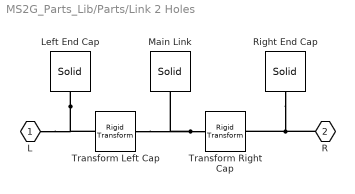
== system MS2G_Parts_Lib/Parts/Link 2 Holes ==
  Left End Cap : sm_lib/Body Elements/Solid  InertiaType=CalculateFromGeometry  Mass=1  MassUnits=kg  CenterOfMass=[0 0 0]  CenterOfMassUnits=m  MomentsOfInertia=[1 1 1]  MomentsOfInertiaUnits=kg*m^2  ProductsOfInertia=[0 0 0]  ProductsOfInertiaUnits=kg*m^2  DensityBased=on  Density=rho  DensityUnits=kg/m^3  DoExposeReferenceFrame=on  SerializedFrames=<Frames/>  GraphicType=FromGeometry  MarkerShape=Sphere  MarkerSize=1  MarkerSizeUnits=m  GraphicVisPropType=SimpleVisualProperties  GraphicDiffuseColor=clr  GraphicSpecularColor=[0.2 0.2 0.2]  GraphicAmbientColor=[0.5 0.5 0.5]  GraphicEmissiveColor=[0.1 0.1 0.1]  GraphicShininess=24.0  GraphicOpacity=opc  GeometryShape=GeneralExtrusion  RectangleSize=[1 1]  RectangleSizeUnits=m  BrickDimensions=[1 1 1]  BrickDimensionUnits=m  CylinderRadius=1  CylinderRadiusUnits=m  CylinderLength=1  CylinderLengthUnits=m  SphereRadius=1  SphereRadiusUnits=m  EllipsoidRadii=[1 1 1]  EllipsoidRadiiUnits=m  ExtrusionCrossSection=Extr_Data_Ring(W/2,r,90,270)  ExtrusionCrossSectionUnits=cm  ExtrusionLength=T  ExtrusionLengthUnits=cm  PolygonNumSides=1  PolygonOuterRadius=1  PolygonOuterRadiusUnits=m  ExtGeomFileType=STEP  ExtGeomFileUnits=m  RevolutionCrossSection=[1 1; 1 -1; 2 -1; 2 1]  RevolutionCrossSectionUnits=m  RevolutionExtent=Full  RevolutionAngle=180  RevolutionAngleUnits=deg
  Main Link : sm_lib/Body Elements/Solid  InertiaType=CalculateFromGeometry  Mass=1  MassUnits=kg  CenterOfMass=[0 0 0]  CenterOfMassUnits=m  MomentsOfInertia=[1 1 1]  MomentsOfInertiaUnits=kg*m^2  ProductsOfInertia=[0 0 0]  ProductsOfInertiaUnits=kg*m^2  DensityBased=on  Density=rho  DensityUnits=kg/m^3  DoExposeReferenceFrame=on  SerializedFrames=<Frames/>  GraphicType=FromGeometry  MarkerShape=Sphere  MarkerSize=1  MarkerSizeUnits=m  GraphicVisPropType=SimpleVisualProperties  GraphicDiffuseColor=clr  GraphicSpecularColor=[0.2 0.2 0.2]  GraphicAmbientColor=[0.5 0.5 0.5]  GraphicEmissiveColor=[0.1 0.1 0.1]  GraphicShininess=24.0  GraphicOpacity=opc  GeometryShape=GeneralExtrusion  RectangleSize=[1 1]  RectangleSizeUnits=m  BrickDimensions=[1 1 1]  BrickDimensionUnits=m  CylinderRadius=1  CylinderRadiusUnits=m  CylinderLength=1  CylinderLengthUnits=m  SphereRadius=1  SphereRadiusUnits=m  EllipsoidRadii=[1 1 1]  EllipsoidRadiiUnits=m  ExtrusionCrossSection=Extr_Data_Link2Hole(L,W,r)  ExtrusionCrossSectionUnits=cm  ExtrusionLength=T  ExtrusionLengthUnits=cm  PolygonNumSides=1  PolygonOuterRadius=1  PolygonOuterRadiusUnits=m  ExtGeomFileType=STEP  ExtGeomFileUnits=m  RevolutionCrossSection=[1 1; 1 -1; 2 -1; 2 1]  RevolutionCrossSectionUnits=m  RevolutionExtent=Full  RevolutionAngle=180  RevolutionAngleUnits=deg
  Right End Cap : sm_lib/Body Elements/Solid  InertiaType=CalculateFromGeometry  Mass=1  MassUnits=kg  CenterOfMass=[0 0 0]  CenterOfMassUnits=m  MomentsOfInertia=[1 1 1]  MomentsOfInertiaUnits=kg*m^2  ProductsOfInertia=[0 0 0]  ProductsOfInertiaUnits=kg*m^2  DensityBased=on  Density=rho  DensityUnits=kg/m^3  DoExposeReferenceFrame=on  SerializedFrames=<Frames/>  GraphicType=FromGeometry  MarkerShape=Sphere  MarkerSize=1  MarkerSizeUnits=m  GraphicVisPropType=SimpleVisualProperties  GraphicDiffuseColor=clr  GraphicSpecularColor=[0.2 0.2 0.2]  GraphicAmbientColor=[0.5 0.5 0.5]  GraphicEmissiveColor=[0.1 0.1 0.1]  GraphicShininess=24.0  GraphicOpacity=opc  GeometryShape=GeneralExtrusion  RectangleSize=[1 1]  RectangleSizeUnits=m  BrickDimensions=[1 1 1]  BrickDimensionUnits=m  CylinderRadius=1  CylinderRadiusUnits=m  CylinderLength=1  CylinderLengthUnits=m  SphereRadius=1  SphereRadiusUnits=m  EllipsoidRadii=[1 1 1]  EllipsoidRadiiUnits=m  ExtrusionCrossSection=Extr_Data_Ring(W/2,r,-90,90)  ExtrusionCrossSectionUnits=cm  ExtrusionLength=T  ExtrusionLengthUnits=cm  PolygonNumSides=1  PolygonOuterRadius=1  PolygonOuterRadiusUnits=m  ExtGeomFileType=STEP  ExtGeomFileUnits=m  RevolutionCrossSection=[1 1; 1 -1; 2 -1; 2 1]  RevolutionCrossSectionUnits=m  RevolutionExtent=Full  RevolutionAngle=180  RevolutionAngleUnits=deg
  Transform Left Cap : sm_lib/Frames and Transforms/Rigid Transform  TranslationMethod=StandardAxis  TranslationLengthUnit=cm  TranslationStandardAxis=-X  TranslationStandardOffset=L/2  TranslationCartesianOffset=[0 0 0]  TranslationROffset=0  TranslationROffsetUnits=m  TranslationZOffset=0  TranslationZOffsetUnits=m  TranslationThetaOffset=0  TranslationThetaOffsetUnits=deg  RotationMethod=None  RotationAngleUnits=deg  RotationStandardAxis=+Z  RotationAngle=0  RotationArbitraryAxis=[0 0 1]  FollAlignAxisA=+X  BaseAlignAxisA=+Y  FollAlignAxisB=+Y  BaseAlignAxisB=+Z  RotationSequenceAxes=FollowerAxes  RotationSequence=XYX  RotationSequenceAngles=[0 0 0]  RotationSequenceAnglesUnits=deg  RotationMatrix=[1 0 0; 0 1 0; 0 0 1]
  Transform Right Cap : sm_lib/Frames and Transforms/Rigid Transform  TranslationMethod=StandardAxis  TranslationLengthUnit=cm  TranslationStandardAxis=+X  TranslationStandardOffset=L/2  TranslationCartesianOffset=[0 0 0]  TranslationROffset=0  TranslationROffsetUnits=m  TranslationZOffset=0  TranslationZOffsetUnits=m  TranslationThetaOffset=0  TranslationThetaOffsetUnits=deg  RotationMethod=None  RotationAngleUnits=deg  RotationStandardAxis=+Z  RotationAngle=0  RotationArbitraryAxis=[0 0 1]  FollAlignAxisA=+X  BaseAlignAxisA=+Y  FollAlignAxisB=+Y  BaseAlignAxisB=+Z  RotationSequenceAxes=FollowerAxes  RotationSequence=XYX  RotationSequenceAngles=[0 0 0]  RotationSequenceAnglesUnits=deg  RotationMatrix=[1 0 0; 0 1 0; 0 0 1]
  L : PMIOPort  Port=1  Side=Left
  R : PMIOPort  Port=2  Side=Right
  connections:
  Right End Cap/RConn1 -- Transform Right Cap/RConn1 -- R/RConn1
  Left End Cap/RConn1 -- Transform Left Cap/RConn1 -- L/RConn1
  Transform Right Cap/LConn1 -- Main Link/RConn1 -- Transform Left Cap/LConn1
